simulink model "pid_control"  (R2014b)
settings: Solver=FixedStepDiscrete  StartTime=0.0  StopTime=sim_time  FixedStep=T  MaxStep=1e-4  RelTol=1e-6
values from neighbouring files (symbols this model uses):
  g = 9.8    [cart_table.m]    (also in preview_control_c.m; preview_control_params.m)
  T = 1e-4    (= 0.0001)    [cart_table.m]    (also in preview_control_c.m)
  Zc = 1    [cart_table.m]    (also in preview_control_c.m)
libraries: simulink x1
settings Model: Creator=StipudUser  LastModifiedBy=aelphy
settings SolverCC: AlgebraicLoopSolver=LineSearch

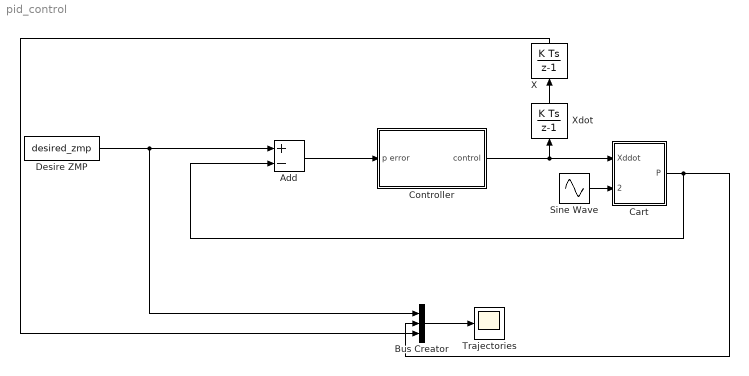
== system pid_control ==
  Add : Sum  Inputs=+-
  Bus Creator : BusCreator  Inputs=3
  Cart : Subsystem
  "Controller " : Subsystem
  "Desire ZMP " : FromWorkspace  VariableName=desired_zmp  SampleTime=T  OutputAfterFinalValue=Setting to zero
  Sine Wave : Sin  Amplitude=0  Bias=Zc  Frequency=2  SampleTime=T
  Trajectories : Scope
      settings: TickLabels=on  ShowLegends=on  TimeRange=10  YMin=0  YMax=1  MaxDataPoints=500000  SampleTime=0.0001
  X : DiscreteIntegrator  SampleTime=-1
  "Xdot " : DiscreteIntegrator  SampleTime=-1
  wires:
  Cart/1("P ") -> Bus Creator/2, Add/2
  Add/1 -> "Controller "/1(p error)
  "Desire ZMP "/1 -> Bus Creator/1, Add/1
  Sine Wave/1 -> Cart/2("Y_CoM ")
  "Controller "/1(control) -> "Xdot "/1, Cart/1("Xddot ")
  "Xdot "/1 -> X/1
  X/1 -> Bus Creator/3
  Bus Creator/1 -> Trajectories/1

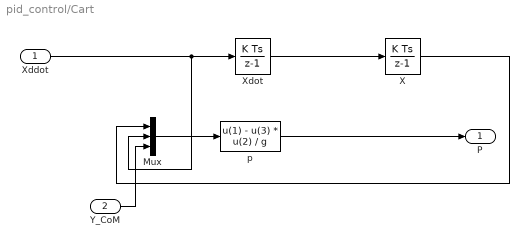
== system pid_control/Cart ==
  "Xddot " : Inport
  "Y_CoM " : Inport  Port=2
  Mux : Mux  Inputs=3
  X : DiscreteIntegrator  SampleTime=-1
  "Xdot " : DiscreteIntegrator  SampleTime=-1
  p : Fcn  Expr=u(1) - u(3) * u(2) / g
  "P " : Outport
  wires:
  p/1 -> "P "/1
  Mux/1 -> p/1
  "Xdot "/1 -> X/1
  X/1 -> Mux/1
  "Y_CoM "/1 -> Mux/3
  "Xddot "/1 -> Mux/2, "Xdot "/1

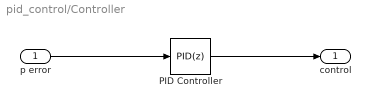
== system pid_control/Controller  ==
  p error : Inport
  PID Controller : simulink/Continuous/PID Controller  Controller=PID  TimeDomain=Discrete-time  SampleTime=-1  IntegratorMethod=Forward Euler  FilterMethod=Forward Euler  Form=Parallel  P=0.315642982555606  I=0.00507784010309176  D=1.49091409547958  N=4.25640184616882  InitialConditionSource=internal  InitialConditionForIntegrator=0  InitialConditionForFilter=0  ExternalReset=none  LimitOutput=off  UpperSaturationLimit=inf  LowerSaturationLimit=-inf  LinearizeAsGain=on  AntiWindupMode=none  Kb=1  TrackingMode=off  Kt=1  PParamMin=[]  PParamMax=[]  IParamMin=[]  IParamMax=[]  DParamMin=[]  DParamMax=[]  NParamMin=[]  NParamMax=[]  KbParamMin=[]  KbParamMax=[]  KtParamMin=[]  KtParamMax=[]  POutMin=[]  POutMax=[]  IOutMin=[]  IOutMax=[]  DOutMin=[]  DOutMax=[]  NOutMin=[]  NOutMax=[]  KbOutMin=[]  KbOutMax=[]  KtOutMin=[]  KtOutMax=[]  IntegratorOutMin=[]  IntegratorOutMax=[]  FilterOutMin=[]  FilterOutMax=[]  SumOutMin=[]  SumOutMax=[]  SumI1OutMin=[]  SumI1OutMax=[]  SumI2OutMin=[]  SumI2OutMax=[]  SumI3OutMin=[]  SumI3OutMax=[]  SumDOutMin=[]  SumDOutMax=[]  SaturationOutMin=[]  SaturationOutMax=[]  IntegratorContinuousStateAttributes=''  IntegratorStateMustResolveToSignalObject=off  IntegratorRTWStateStorageClass=Auto  FilterContinuousStateAttributes=''  FilterStateMustResolveToSignalObject=off  FilterRTWStateStorageClass=Auto  DifferentiatorICPrevScaledInput=0  DifferentiatorOutMin=[]  DifferentiatorOutMax=[]  UseFilter=on
  control : Outport
  wires:
  PID Controller/1 -> control/1
  p error/1 -> PID Controller/1
